simulink model "modelForExperiment"  (R2020b)
settings: Solver=ode5  StartTime=0.0  StopTime=Inf  FixedStep=0.001  RelTol=1e-3
undefined symbols (not defined in the file): A, deltaW, Kd, Ki, Kp, National_Instruments, PCI, rpm2degs, sens, Tl
libraries: sldrtlib x3, simulink x2
settings Model: ExtModeTrigDuration=100000  Creator=umbe  LastModifiedBy=castiumber
settings RTWCC: Description=Simulink Desktop Real-Time  SystemTargetFile=sldrt.tlc  TemplateMakefile=sldrt.tmf  RTWCompilerOptimization=on
settings CodeAppCC: MaxIdLength=95
settings SimulinkDesktopRealTimeCC: TargetPreCompLibLocation=C:\Program Files\MATLAB\R2020b\toolbox\sldrt\lib\win64

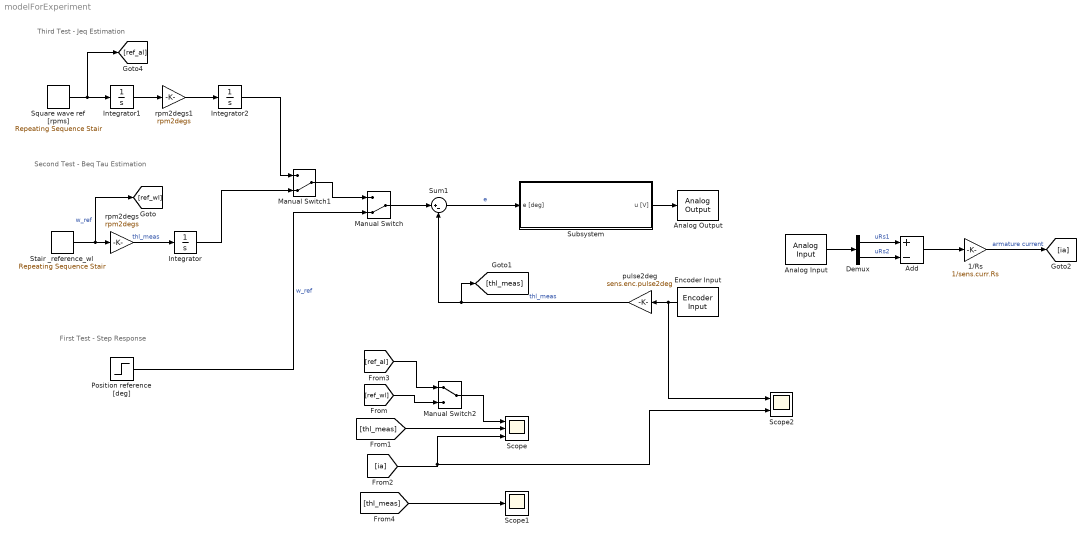
== system modelForExperiment ==
  note: Third Test - Jeq Estimation
  note: Second Test - Beq Tau Estimation
  note: First Test - Step Response
  1/Rs : Gain  Gain=1/sens.curr.Rs
  Add : Sum  Inputs=+-
  Analog Input : sldrtlib/Analog Input  SampleTime=0.001  MaxMissedTicks=10  ShowMissedTicks=off  YieldWhenWaiting=off  DrvName=National_Instruments/PCI-6221  DrvAddress=4294967295  DrvOptions=[0 0 0 2 0]  Channels=[1 2]  RangeMode=1  VoltRange=1  DataType=1
      settings: AttributesFormatString=National Instruments\nPCI-6221 [auto]
  Analog Output : sldrtlib/Analog Output  SampleTime=0.001  MaxMissedTicks=10  ShowMissedTicks=off  YieldWhenWaiting=off  DrvName=National_Instruments/PCI-6221  DrvAddress=4294967295  DrvOptions=[0 0 0 2 0]  Channels=1  RangeMode=1  VoltRange=1  InitialValue=0  FinalValue=0
      settings: AttributesFormatString=National Instruments\nPCI-6221 [auto]
  Demux : Demux  Outputs=2
  Encoder Input : sldrtlib/Encoder Input  SampleTime=0.001  MaxMissedTicks=10  ShowMissedTicks=off  YieldWhenWaiting=off  DrvName=National_Instruments/PCI-6221  DrvAddress=4294967295  DrvOptions=[0 0 0 2 0]  Channels=1  QuadMode=3  IndexPulse=1  InputFilter=Inf  DataType=1
      settings: AttributesFormatString=National Instruments\nPCI-6221 [auto]
  Integrator : Integrator
  Integrator1 : Integrator
  Integrator2 : Integrator
  Manual Switch : ManualSwitch  CurrentSetting=0
  Manual Switch1 : ManualSwitch  CurrentSetting=0
  Manual Switch2 : ManualSwitch
  Position reference [deg] : Step  After=10  SampleTime=0
  Scope : Scope  NumInputPorts=3
  Scope1 : Scope
  Scope2 : Scope  NumInputPorts=2
  Square wave ref [rpms] : simulink/Sources/Repeating Sequence Stair  OutValues=A*[1 -1].'  tsamp=deltaTAcc  OutMin=[]  OutMax=[]  OutDataTypeStr=double  OutputDataTypeScalingMode=double  OutDataType=fixdt(0,8)  ConRadixGroup=Best Precision: Vector-wise  OutScaling=2^-12
  Stair _reference_wl : simulink/Sources/Repeating Sequence Stair  OutValues=-deltaW*[1 2 3 4 5 6 7 8 9 9].'  tsamp=deltaT  OutMin=[]  OutMax=[]  OutDataTypeStr=double  OutputDataTypeScalingMode=double  OutDataType=fixdt(0,8)  ConRadixGroup=Best Precision: Vector-wise  OutScaling=2^-12
  Subsystem : Subsystem
  Sum1 : Sum  Inputs=|+-
  pulse2deg : Gain  Gain=sens.enc.pulse2deg
  rpm2degs : Gain  Gain=rpm2degs
  rpm2degs1 : Gain  Gain=rpm2degs
  wires:
  1/Rs/1 -> [ia]  "armature current"
  Add/1 -> 1/Rs/1
  Demux/1 -> Add/1  "uRs1"
  Demux/2 -> Add/2  "uRs2"
  pulse2deg/1 -> [thl_meas], Sum1/2  "thl_meas"
  Sum1/1 -> Subsystem/1(e [deg])  "e"
  Stair _reference_wl/1 -> [ref_wl], rpm2degs/1  "w_ref"
  Integrator/1 -> Manual Switch1/2
  Manual Switch/1 -> Sum1/1
  [ref_wl] -> Manual Switch2/2
  [thl_meas] -> Scope/2
  [ia] -> Scope2/2, Scope/3
  rpm2degs/1 -> Integrator/1  "thl_meas"
  Integrator2/1 -> Manual Switch1/1
  rpm2degs1/1 -> Integrator2/1
  Integrator1/1 -> rpm2degs1/1
  Square wave ref [rpms]/1 -> [ref_al], Integrator1/1
  Manual Switch2/1 -> Scope/1
  [ref_al] -> Manual Switch2/1
  Manual Switch1/1 -> Manual Switch/1
  [thl_meas] -> Scope1/1
  Encoder Input/1 -> Scope2/1, pulse2deg/1
  Analog Input/1 -> Demux/1
  Subsystem/1(u [V]) -> Analog Output/1
  Position reference [deg]/1 -> Manual Switch/2  "w_ref"

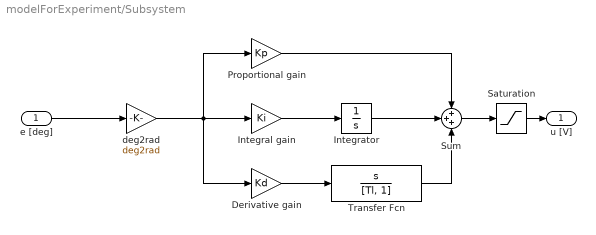
== system modelForExperiment/Subsystem ==
  e [deg] : Inport
  Derivative gain : Gain  Gain=Kd
  Integral gain : Gain  Gain=Ki
  Integrator : Integrator
  Proportional gain : Gain  Gain=Kp
  Saturation : Saturate  UpperLimit=10  LowerLimit=-10
  Sum : Sum  Inputs=+++
  Transfer Fcn : TransferFcn  Numerator=[1,0]  Denominator=[Tl, 1]
  deg2rad : Gain  Gain=deg2rad
  u [V] : Outport
  wires:
  Transfer Fcn/1 -> Sum/3
  Integrator/1 -> Sum/2
  e [deg]/1 -> deg2rad/1
  deg2rad/1 -> Integral gain/1, Proportional gain/1, Derivative gain/1
  Saturation/1 -> u [V]/1
  Derivative gain/1 -> Transfer Fcn/1
  Sum/1 -> Saturation/1
  Integral gain/1 -> Integrator/1
  Proportional gain/1 -> Sum/1
